simulink model "AD9144"  (R2014b)
settings: Solver=FixedStepDiscrete  StartTime=0.0  StopTime=StopTime  FixedStep=1/Fdac  RelTol=1e-3
InitFcn:
  | % Globals
  | NLength = 2^12;
  | Tessitura = 130e6; % Input Frequency
  | L = 2;   % Interpolation: {1,2,4,8}
  | Res = 16;
  | Fdac = 2120e6;
  | 
  | % Calculations
  | Fdata = min(Fdac / L, 1060e6);
  | Samples_per_second = round(1/(Tessitura/Fdata));
  | N_offset_samples = Samples_per_second / 4;
  | 
  | StopTime = NLength / Fdata;
undefined symbols (not defined in the file or in its folder): tessitura
settings Model: Creator=tmacleod  LastModifiedBy=tmacleod
settings SolverCC: AutoInsertRateTranBlk=on

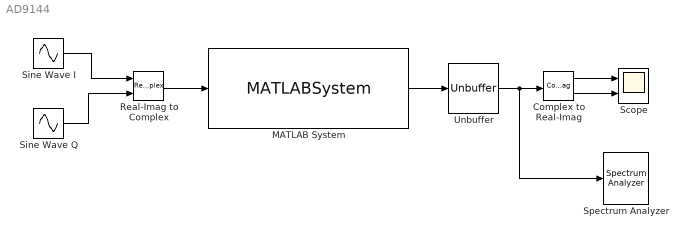
== system AD9144 ==
  Complex to Real-Imag : ComplexToRealImag
  MATLAB System : MATLABSystem  System=AD9144_sysobj  SimulateUsing=Interpreted execution  Mode=Nominal  Interpolation=L  Fdata=Fdata  NcoFreq=0  InvSinc=Disabled  OutputConfig=Normalized
      mask Type: AD9144_sysobj
      mask Display:
      | disp('AD9144');
      | port_label('input',1,'in (Code)');
      | port_label('output',1,'out (A)');
  Real-Imag to Complex : RealImagToComplex
  Scope : Scope  NumInputPorts=2
      settings: YMin=-5~-5  YMax=5~5
  Sine Wave I : Sin  SineType=Sample based  Amplitude=2^(Res-1)  Bias=2^(Res-1)  Frequency=2*pi*tessitura  Samples=Samples_per_second  SampleTime=1/Fdata
  Sine Wave Q : Sin  SineType=Sample based  Amplitude=2^(Res-1)  Bias=2^(Res-1)  Frequency=2*pi*tessitura  Phase=-pi/2  Samples=Samples_per_second  SampleTime=1/Fdata  Offset=N_offset_samples
  Spectrum Analyzer : SpectrumAnalyzer
  Unbuffer : Unbuffer  SampleBasedProcessing=Same as frame based
  wires:
  Complex to Real-Imag/1 -> Scope/1
  Complex to Real-Imag/2 -> Scope/2
  Sine Wave I/1 -> Real-Imag to Complex/1
  Sine Wave Q/1 -> Real-Imag to Complex/2
  Real-Imag to Complex/1 -> MATLAB System/1
  MATLAB System/1 -> Unbuffer/1
  Unbuffer/1 -> Spectrum Analyzer/1, Complex to Real-Imag/1
